simulink model "Pen_inv_Controlador_observador"  (R2020b)
settings: Solver=VariableStepAuto  StartTime=0.0  StopTime=20  FixedStep=1e-6  RelTol=1e-3
settings Model: Creator=Marce  LastModifiedBy=Marce

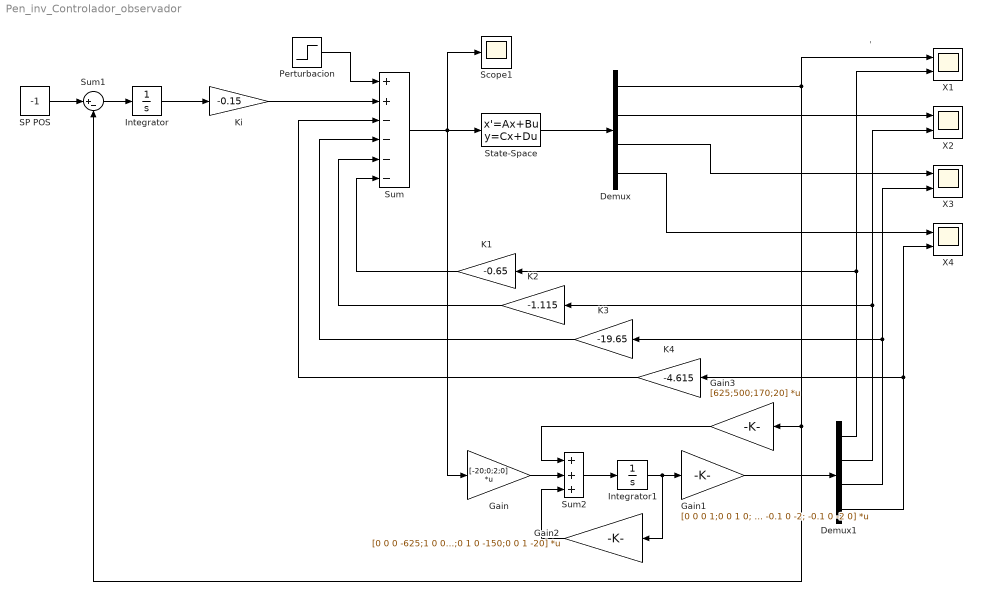
== system Pen_inv_Controlador_observador ==
  note: '
  Demux : Demux
  Demux1 : Demux
  Gain : Gain  Gain=[-20;0;2;0]  Multiplication=Matrix(K*u)
  Gain1 : Gain  Gain=[0 0 0 1;0 0 1 0; 0 -0.1 0 -2; -0.1 0 -2 0]  Multiplication=Matrix(K*u) (u vector)
  Gain2 : Gain  Gain=[0 0 0 -625;1 0 0 -500;0 1 0 -150;0 0 1 -20]  Multiplication=Matrix(K*u) (u vector)
  Gain3 : Gain  Gain=[625;500;170;20]  Multiplication=Matrix(K*u)
  Integrator : Integrator
  Integrator1 : Integrator  InitialCondition=[0;0;0;0]
  K1 : Gain  Gain=-0.65
  K2 : Gain  Gain=-1.115
  K3 : Gain  Gain=-19.65
  K4 : Gain  Gain=-4.615
  Ki : Gain  Gain=-0.15
  Perturbacion : Step  Time=7  After=0.5  SampleTime=0
  SP POS : Constant  Value=-1
  Scope1 : Scope
  State-Space : StateSpace  A=[0 1 0 0;0 0 -10 0;0 0 0 1;0 0 20 0]  B=[0;2;0;-2]  C=[1 0 0 0;0 1 0 0;0 0 1 0;0 0 0 1]  D=[0;0;0;0]  InitialCondition=[0.5;0.2; 0.1;0.01]
  Sum : Sum  Inputs=++----
  Sum1 : Sum  Inputs=|+-
  Sum2 : Sum  Inputs=+++
  X{1..4} (4 alike) : Scope  NumInputPorts=2
  wires:
  SP POS/1 -> Sum1/1
  Sum1/1 -> Integrator/1
  Integrator/1 -> Ki/1
  Ki/1 -> Sum/2
  Sum/1 -> Gain/1, Scope1/1, State-Space/1
  Perturbacion/1 -> Sum/1
  Gain/1 -> Sum2/2
  Gain3/1 -> Sum2/1
  State-Space/1 -> Demux/1
  Gain2/1 -> Sum2/3
  Integrator1/1 -> Gain2/1, Gain1/1
  Sum2/1 -> Integrator1/1
  Gain1/1 -> Demux1/1
  Demux/2 -> X2/1
  Demux1/2 -> X2/2, K2/1
  Demux1/3 -> K3/1, X3/2
  Demux/3 -> X3/1
  Demux1/4 -> K4/1, X4/2
  Demux/4 -> X4/1
  K4/1 -> Sum/3
  K3/1 -> Sum/4
  K2/1 -> Sum/5
  K1/1 -> Sum/6
  Demux1/1 -> K1/1, X1/2
  Demux/1 -> Gain3/1, Sum1/2, X1/1
